simulink model "ElevePuissanceLampe"  (R2018a)
settings: Solver=VariableStepAuto  StartTime=0.0  StopTime=inf  RelTol=1e-3  EnableMultiTasking=on
settings Model: Creator=djellal  LastModifiedBy=poingt
settings DataIOCC: LimitDataPoints=on
settings OptimizationCC: LifeSpan=inf
settings DebuggingCC: AllowSymbolicDim=off  SFUnexpectedBacktrackingDiag=warning  SFNoUnconditionalDefaultTransitionDiag=warning  SFExecutionAtInitializationDiag=none
settings ModelReferenceCC: PropagateSignalLabelsOutOfModel=off
settings CodeAppCC: StateflowObjectComments=on
settings GRTTargetCC: TargetLangStandard=C89/C90 (ANSI)
settings ConfigComp: CovMetricSettings=dw  CovHtmlReporting=on  CovSaveCumulativeToWorkspaceVar=on  CovSaveSingleToWorkspaceVar=on  CovExternalEMLEnable=off
settings SimscapeCC: SimscapeNormalizeSystem=off
settings SimMechanicsCC: VisOnUpdateDiagram=on  VisDuringSimulation=on
settings ConfigurationSet: Description=SimMechanics 2G

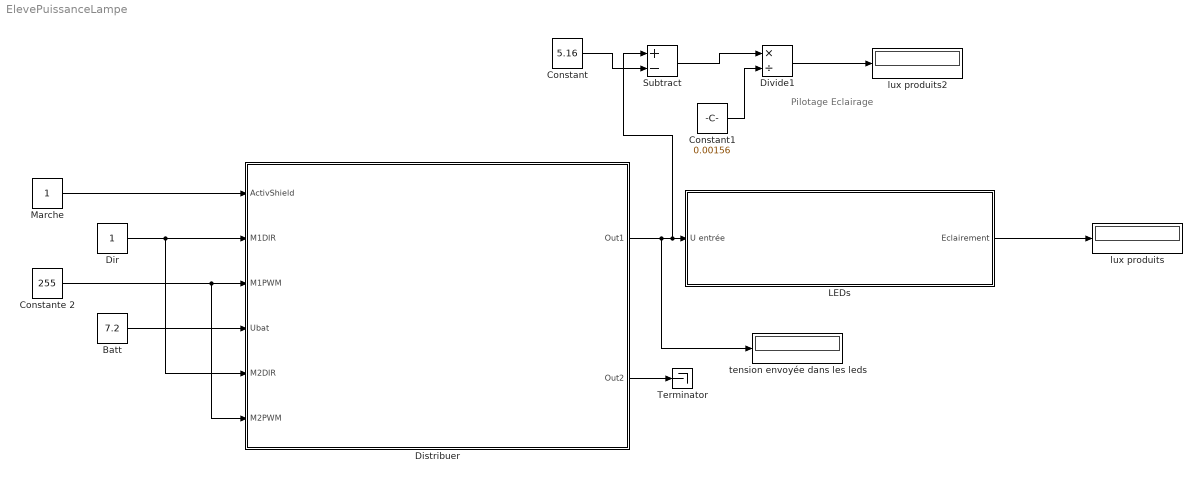
== system ElevePuissanceLampe ==
  note: Pilotage Eclairage
  Batt : Constant  Value=7.2  SampleTime=5
  Constant : Constant  Value=5.16
  Constant1 : Constant  Value=0.00156
  Constante 2 : Constant  Value=255
  Dir : Constant
  Distribuer : Subsystem
      mask Display:
      | image(imread('shieldMC33926.jpg'))
      | port_label('output', 1, 'Ushld1')
      | port_label('output', 2, 'Ushld2')
      | port_label('input', 1, 'Active')
      | port_label('input', 2, 'Dir1')
      | port_label('input', 3, 'PWM1')
      | port_label('input', 4, 'Ualim')
      | port_label('input', 5, 'Dir2')
      | port_label('input', 6, 'PWM2')
  Divide1 : Product  Inputs=*/
  LEDs : Subsystem  mask{Vmin=5, P=7.2*0.06, Vmax=7.2}
      mask prompts: Vmin "Tension minimale (V)"; P "Puissance (W)"; Vmax "Tension maximale"
      mask Display:
      | image(imread('led.jpg'))
      | port_label('input', 1, 'U')
      | port_label('output', 1, 'Eclairement')
  "Marche " : Constant
  Subtract : Sum  Inputs=+-
  Terminator : Terminator
  lux produits : Display
  lux produits2 : Display
  tension envoyée dans les leds : Display
  wires:
  Batt/1 -> Distribuer/4(Ubat)
  "Marche "/1 -> Distribuer/1(ActivShield)
  Dir/1 -> Distribuer/2(M1DIR), Distribuer/5("M2DIR ")
  Distribuer/1(Out1) -> tension envoyée dans les leds/1, Subtract/1, LEDs/1(U entrée)
  Constante 2/1 -> Distribuer/6(M2PWM), Distribuer/3(M1PWM)
  Distribuer/2(Out2) -> Terminator/1
  LEDs/1(Eclairement) -> lux produits/1
  Constant/1 -> Subtract/2
  Subtract/1 -> Divide1/1
  Constant1/1 -> Divide1/2
  Divide1/1 -> lux produits2/1

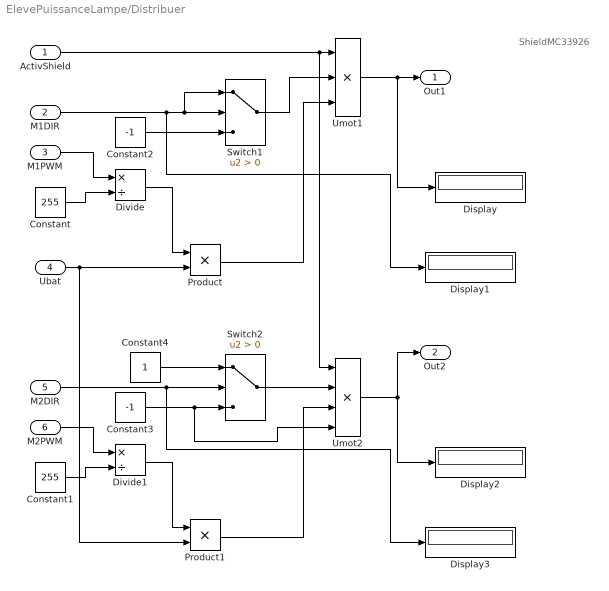
== system ElevePuissanceLampe/Distribuer ==
  note: ShieldMC33926
  ActivShield : Inport
  M1DIR : Inport  Port=2
  M1PWM : Inport  Port=3
  Ubat : Inport  Port=4
  "M2DIR " : Inport  Port=5
  M2PWM : Inport  Port=6
  Constant : Constant  Value=255
  Constant1 : Constant  Value=255
  Constant2 : Constant  Value=-1
  Constant3 : Constant  Value=-1
  Constant4 : Constant
  Display{,1..3} (4 alike) : Display
  Divide : Product  Inputs=*/
  Divide1 : Product  Inputs=*/
  Product : Product
  Product1 : Product
  Switch1 : Switch  Criteria=u2 > Threshold
  Switch2 : Switch  Criteria=u2 > Threshold
  Umot1 : Product  Inputs=3
  Umot2 : Product  Inputs=4
  Out1 : Outport
  Out2 : Outport  Port=2
  wires:
  Ubat/1 -> Product1/2, Product/2
  M1PWM/1 -> Divide/1
  Constant/1 -> Divide/2
  Divide/1 -> Product/1
  Umot1/1 -> Display/1, Out1/1
  Product/1 -> Umot1/3
  M1DIR/1 -> Display1/1, Switch1/2, Switch1/1
  Constant2/1 -> Switch1/3
  Switch1/1 -> Umot1/2
  ActivShield/1 -> Umot2/1, Umot1/1
  M2PWM/1 -> Divide1/1
  Constant1/1 -> Divide1/2
  Divide1/1 -> Product1/1
  Umot2/1 -> Out2/1, Display2/1
  Product1/1 -> Umot2/3
  "M2DIR "/1 -> Display3/1, Switch2/2
  Constant3/1 -> Umot2/4, Switch2/3
  Switch2/1 -> Umot2/2
  Constant4/1 -> Switch2/1

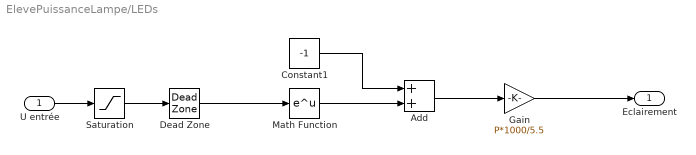
== system ElevePuissanceLampe/LEDs ==
  U entrée : Inport
  Add : Sum
  Constant1 : Constant  Value=-1
  Dead Zone : DeadZone  LowerValue=0  UpperValue=Vmin  SaturateOnIntegerOverflow=on
  Gain : Gain  Gain=P*1000/5.5
  Math Function : Math  SaturateOnIntegerOverflow=on
  Saturation : Saturate  UpperLimit=Vmax  LowerLimit=0
  Eclairement : Outport
  wires:
  U entrée/1 -> Saturation/1
  Dead Zone/1 -> Math Function/1
  Math Function/1 -> Add/2
  Constant1/1 -> Add/1
  Add/1 -> Gain/1
  Gain/1 -> Eclairement/1
  Saturation/1 -> Dead Zone/1
